simulink model "RBFNN_1221"  (R2018a)
settings: Solver=FixedStepAuto  StartTime=0.0  StopTime=inf  FixedStep=0.001  RelTol=1e-3  EnableMultiTasking=on
undefined symbols (not defined in the file): HIL, j, qc_get_step_size
libraries: dsparch4 x28, quarc_library x17, simulink x7, vrlib x1
(part 6 of 6)

== matlab function RBFNN_1221/RBFNN_wrist1 ==
  data: W_F input; W_Q input; U_F output; U_Q output; z1 input; z2 input; W_F_next output; W_Q_next output; W_F_dot output; z3 input; p1 input; p2 input; qd input; qd_dot input; qd_ddot input; gamma_NN_F input; gamma_NN_Q input; eta_F input; eta_Q input; look output
function [U_F, U_Q, W_F_next, W_Q_next, W_F_dot, look] = RBFNN(W_F, W_Q, z1, z2, z3, p1, p2, qd, qd_dot, qd_ddot, gamma_NN_F, gamma_NN_Q, eta_F, eta_Q)

% 仿真环境
ts = 0.0002;

%-------控制器需输入信息--------

% RBFNN控制参数

%手腕关节中心点参数
cij= [-0.499106221625804, -0.499106221625804,  2005.79872399738,  2639144.26212096,  2223202.48890840,  -0.493324863755757,  -0.0232163020531828,   0.127650732846403;
      -1.12620134740565,  -1.12620134740565,   2952.38958819554,  4234769.00352520,  2070148.36236487,  0.196658457787049,  0.0133039268692362,     -0.0826238790945131;
      -1.11695482722882,  -1.11695482722882,   3165.28189098781,  3836085.68692222,  1999734.92258975,  0.153237256316932,  0.0767773705194676,     -0.369349406570774;
      -1.05951865103650,  -1.05951865103650,   3414.12364345425,  3393273.20854046,  2007071.20329101,  -0.0589190714477196,  0.00750783405961825,  -0.229262334963137;
      -0.694285708154741, -0.694285708154741,  2654.85166253362,  2956383.72448738,  2078438.60445473,  -0.376420334916739,  -0.0230368382437097,   -0.57526;]';
b = 7e6;                                                                                          
% cij = [-0.439933888449828,-0.439933888449828,2451.55347804672,2767814.47175142,2176437.85549850,-0.496782422951389,-0.0218399547939797,0.0992537523291070;
%     -0.707091945857437,-0.707091945857437,-1201.30499796279,4105011.96443656,2307085.59595542,0.195229208102849,0.0212397964660078,-0.104118523361863;
%     -0.482080296325197,-0.482080296325197,2482.99966383581,3064346.25915951,2214695.93802147,-0.419640215636631,-0.0667932707214427,0.417784591553494;
%     -0.621099857750493,-0.621099857750493,-1955.03858922138,3423743.69626516,2244963.95661695,-0.122370078655306,-0.0111107223090986,-0.0596028618004376;
%     -0.626015628808877,-0.626015628808877,1307.10684650810,3777242.51334384,2276658.90151799,0.135342448786687,0.0865881830302452,-0.380789397425015;]';

% cij = zeros(8,5,2);
% cij(:,:,1) = cij_wrist; cij(:,:,2) = cij_smallarm;

row = size(cij,2);
% 同样对z3, p1, p2处理
x_input = [z1; z2; z3; p1; p2; qd; qd_dot; qd_ddot];
h = zeros(row,1); 

W_F_dot = zeros(row,1);
W_Q_dot = zeros(row,1);
for j = 1:1:row
    h(j) = exp(-norm(x_input-cij(:,j))^2/(b^2));
    W_F_dot(j) = gamma_NN_F * (z2 * h(j) - eta_F  * W_F(j));
    W_Q_dot(j) = gamma_NN_Q * (z3 * h(j)- eta_Q  * W_Q(j));
    W_F_dot(j) = gamma_NN_F * (z2 * h(j) - eta_F * abs(z2) * W_F(j));
    W_Q_dot(j) = gamma_NN_Q * (z3 * h(j)- eta_Q * abs(z3) * W_Q(j));
    %限制幅值
    W_F_dot(j) = min(max(W_F_dot(j), -500), 500);
    W_Q_dot(j) = min(max(W_Q_dot(j), -1e-5), 1e-5);
end




W_F_next = W_F_dot * ts + W_F;
W_Q_next = W_Q_dot * ts + W_Q;
%-------Output--------
RBFNN_F = W_F'*h;                                                               % 控制器输出电压
RBFNN_Q = W_Q'*h;  
% RBFNN_F = min(max(RBFNN_F, -100), 100);
% % RBFNN_Q = min(max(RBFNN_Q, -1e-5), 1e-4);
U_F = RBFNN_F*200;
U_Q = RBFNN_Q;
look  = W_F;
